simulink model "OFDM_QAM_256"  (R2017a)
settings: Solver=VariableStepAuto  StartTime=0.0  StopTime=3*1/15e3  RelTol=1e-3
model workspace (MAT data in the model file):
  M = 64
libraries: dspxfrm3 x2, dspspect3 x2, dspindex x2, commdigbbndam3 x2, dspsnks4 x2, commchan3 x1, commsink2 x1, commrandsrc2 x1
settings Model: Creator=Sommc  LastModifiedBy=romainsercer

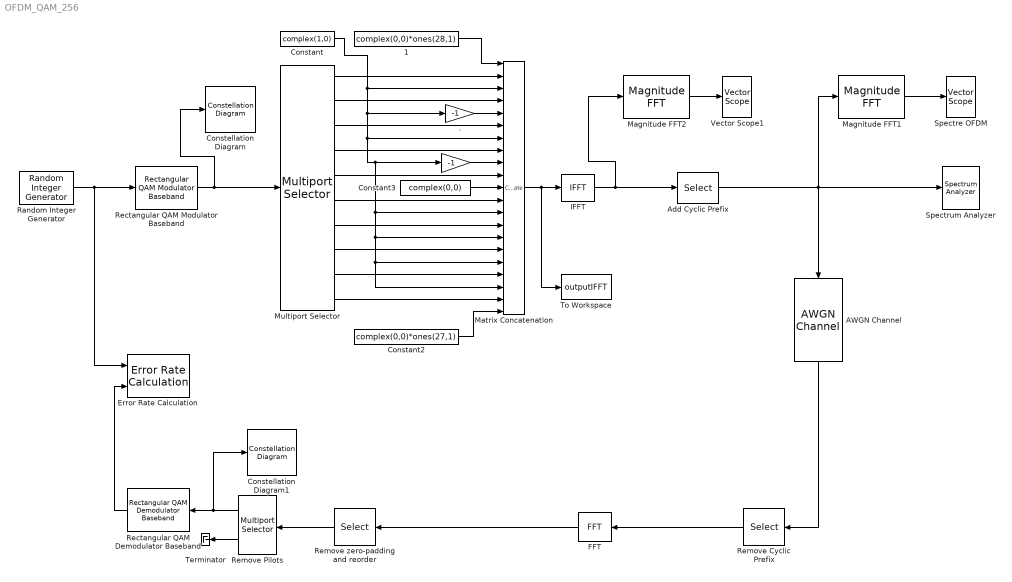
== system OFDM_QAM_256 ==
  " " : Gain  Gain=-1
  " 1" : Constant  Value=complex(0,0)*ones(28,1)
  . : Gain  Gain=-1
  AWGN Channel : commchan3/AWGN Channel  InputProcessing=Inherited (this choice will be removed - see release notes)  seed=34  noiseMode="Signal to noise ratio  (SNR)"  EbNodB=10  EsNodB=10  SNRdB=snr  bitsPerSym=1  Ps=0.01  Tsym=1  variance=1
  Add Cyclic Prefix : Selector  InputPortWidth=256  IndexOptions=Index vector (dialog)  Indices=[193:256 1:256]  OutputSizes=[(-2)]
  Constant : Constant  Value=complex(1,0)
  Constant2 : Constant  Value=complex(0,0)*ones(27,1)
  Constant3 : Constant  Value=complex(0,0)
  Constellation Diagram : ConstellationDiagram
  Constellation Diagram1 : ConstellationDiagram
  Error Rate Calculation : commsink2/Error Rate Calculation  N=0  st_delay=0  cp_mode=Entire frame  subframe=[]  PMode=Workspace  WsName=value_BER  RsMode2=off  stop=off  numErr=100  maxBits=1e6
  FFT : dspxfrm3/FFT  FFTImplementation=Auto  CompMethod=Table lookup  TableOpt=HYBRID  TableOptActive=Speed  BitRevOrder=off  Normalize=off  InheritFFTLength=on  FFTLength=64  WrapInput=on  roundingMode=Floor  overflowMode=off  firstCoeffDataTypeStr=Inherit: Same word length as input  firstCoeffLastDataTypeStr=Inherit: Same word length as input  outputMin=[]  outputMax=[]
  IFFT : dspxfrm3/IFFT  FFTImplementation=Auto  CompMethod=Table lookup  TableOpt=HYBRID  TableOptActive=Speed  BitRevOrder=off  cs_in=off  Normalize=on  InheritFFTLength=on  FFTLength=64  WrapInput=on  mode=Complex  outSamplingMode=Frame based  roundingMode=Floor  overflowMode=off  firstCoeffDataTypeStr=Inherit: Same word length as input  firstCoeffLastDataTypeStr=Inherit: Same word length as input  outputMin=[]  outputMax=[]
      settings: SourceProductName=DSP System Toolbox
  Magnitude FFT1 : dspspect3/Magnitude FFT  mag_or_magsq=Magnitude  FFTImplementation=Auto  fftLenInherit=off  fftsize=320  WrapInput=on
      settings: SourceProductName=DSP System Toolbox  SourceProductBaseCode=DS
  Magnitude FFT2 : dspspect3/Magnitude FFT  mag_or_magsq=Magnitude  FFTImplementation=Auto  fftLenInherit=on  fftsize=320  WrapInput=on
      settings: SourceProductName=DSP System Toolbox  SourceProductBaseCode=DS
  Matrix Concatenation : Concatenate  NumInputs=21  Mode=Multidimensional array
  Multiport Selector : dspindex/Multiport Selector  rowsOrCols=Rows  idxCellArray={1:12, 13:36, 37:60, 61:84, 85:96, 97:108, 109:132, 133:156, 157:180, 181:192}  idxErrMode=Clip Index
  Random Integer Generator : commrandsrc2/Random Integer Generator  mul=M  seed=37  Ts=1/20e6  frameBased=on  sampPerFrame=192  orient=off  outDataType=double
  Rectangular QAM Demodulator Baseband : commdigbbndam3/Rectangular QAM Demodulator Baseband  M=M  OutType=Integer  DecType=Hard decision  VarSource=Dialog  Variance=1  Dec=Gray  Mapping=[0:15]  PowType=Min. distance between symbols  MinDist=1  AvgPow=1  PeakPow=1  Ph=0  outDtype1=Inherit via internal rule  outDtype2=Inherit via internal rule  derotateFactorWordLen=16  derotateFactorDataTypeStr=Inherit: Same word length as input  derotateFactorLastDataTypeStr=Inherit: Same word length as input  denormFactorWordLen=16  denormFactorDataTypeStr=Inherit: Same word length as input  denormFactorLastDataTypeStr=Inherit: Same word length as input  prodOutWordLen=32  prodOutOverflowMode=Wrap  prodOutRoundingMode=Floor  prodOutOvFlMode=off  prodOutOvFlModeLastStrValue=off  sumWordLen=32
  Rectangular QAM Modulator Baseband : commdigbbndam3/Rectangular QAM Modulator Baseband  M=M  InType=Integer  Enc=Gray  Mapping=[0:15]  PowType=Min. distance between symbols  MinDist=1  AvgPow=1  PeakPow=1  Ph=0  outDtype=double  outWordLen=16  outUDDataType=sfix(16)  outFracLenMode=Best precision  outFracLen=15  outDataTypeStr=double  outLastDataTypeStr=double
  Remove zero-padding and reorder : Selector  InputPortWidth=256  IndexOptions=Index vector (dialog)  Indices=[29:128 130:229]  OutputSizes=[(-2)]
  Remove Pilots : dspindex/Multiport Selector  rowsOrCols=Rows  idxCellArray={[1:12 14:37 39:62 64:87 89:112 114:137 139:162 164:187 189:200],[13 38 63 88 113 138 163 188]}  idxErrMode=Clip Index
  Remove Cyclic Prefix : Selector  InputPortWidth=320  IndexOptions=Index vector (dialog)  Indices=[65:320]  OutputSizes=[(-2)]
  Spectre OFDM : dspsnks4/Vector Scope  ScopeProperties=on  Domain=Frequency  HorizSpan=1  DisplayProperties=off  AxisGrid=on  Memory=off  FrameNumber=on  AxisLegend=on  AxisZoom=off  OpenScopeAtSimStart=on  OpenScopeImmediately=off  FigPos=[440 378 560 420]  AxisProperties=off  XUnits=Hertz  XRange=[0...Fs]  InheritXIncr=on  XIncr=1  XLabel=Time  XLimit=Auto  XMin=0  XMax=16666666.6667  XStart=0  YUnits=dB  YLabel=Amplitude  LineProperties=off  XAxisParamsVer=6.9
      settings: SourceProductName=DSP System Toolbox  SourceProductBaseCode=DS  YMin=-30  YMax=30
  Spectrum Analyzer : SpectrumAnalyzer
  Terminator : Terminator
  To Workspace : ToWorkspace  VariableName=outputIFFT  SampleTime=-1
  Vector Scope1 : dspsnks4/Vector Scope  ScopeProperties=on  Domain=Frequency  HorizSpan=1  DisplayProperties=off  AxisGrid=on  Memory=off  FrameNumber=on  AxisLegend=on  AxisZoom=off  OpenScopeAtSimStart=on  OpenScopeImmediately=off  FigPos=[440 378 560 420]  AxisProperties=off  XUnits=Hertz  XRange=[0...Fs]  InheritXIncr=on  XIncr=1  XLabel=Time  XLimit=User-defined  XMin=0  XMax=26666666.6667  XStart=0  YUnits=dB  YLabel=Amplitude  LineProperties=off  LineColors=[0 0 1]  XAxisParamsVer=6.9
      settings: SourceProductName=DSP System Toolbox  SourceProductBaseCode=DS  YMin=-100  YMax=10
  wires:
  Random Integer Generator/1 -> Error Rate Calculation/1, Rectangular QAM Modulator Baseband/1
  Matrix Concatenation/1 -> To Workspace/1, IFFT/1
  IFFT/1 -> Add Cyclic Prefix/1, Magnitude FFT2/1
  Constant3/1 -> Matrix Concatenation/11
  " "/1 -> Matrix Concatenation/9
  ./1 -> Matrix Concatenation/5
  Constant2/1 -> Matrix Concatenation/21
  " 1"/1 -> Matrix Concatenation/1
  Constant/1 -> ./1, Matrix Concatenation/17, Matrix Concatenation/19, Matrix Concatenation/15, Matrix Concatenation/13, " "/1, Matrix Concatenation/7, Matrix Concatenation/3
  Multiport Selector/10 -> Matrix Concatenation/20
  Multiport Selector/1 -> Matrix Concatenation/2
  Multiport Selector/2 -> Matrix Concatenation/4
  Multiport Selector/3 -> Matrix Concatenation/6
  Multiport Selector/4 -> Matrix Concatenation/8
  Multiport Selector/5 -> Matrix Concatenation/10
  Multiport Selector/6 -> Matrix Concatenation/12
  Multiport Selector/7 -> Matrix Concatenation/14
  Multiport Selector/8 -> Matrix Concatenation/16
  Multiport Selector/9 -> Matrix Concatenation/18
  Rectangular QAM Modulator Baseband/1 -> Constellation Diagram/1, Multiport Selector/1
  Remove Cyclic Prefix/1 -> FFT/1
  Remove Pilots/2 -> Terminator/1
  Remove Pilots/1 -> Constellation Diagram1/1, Rectangular QAM Demodulator Baseband/1
  Remove zero-padding and reorder/1 -> Remove Pilots/1
  FFT/1 -> Remove zero-padding and reorder/1
  Rectangular QAM Demodulator Baseband/1 -> Error Rate Calculation/2
  Magnitude FFT1/1 -> Spectre OFDM/1
  Magnitude FFT2/1 -> Vector Scope1/1
  Add Cyclic Prefix/1 -> Magnitude FFT1/1, Spectrum Analyzer/1, AWGN Channel/1
  AWGN Channel/1 -> Remove Cyclic Prefix/1
